simulink model "GyroCLIdent"  (R2021b)
settings: Solver=FixedStepAuto  StartTime=0.0  StopTime=t(end)  FixedStep=Ts  RelTol=1e-3
undefined symbols (not defined in the file): params, x0
libraries: cstblocks x2
settings Model: Creator=Patrick  LastModifiedBy=tom
settings SolverCC: AlgebraicLoopSolver=TrustRegion
settings DebuggingCC: SFMachineParentedDataDiag=warning

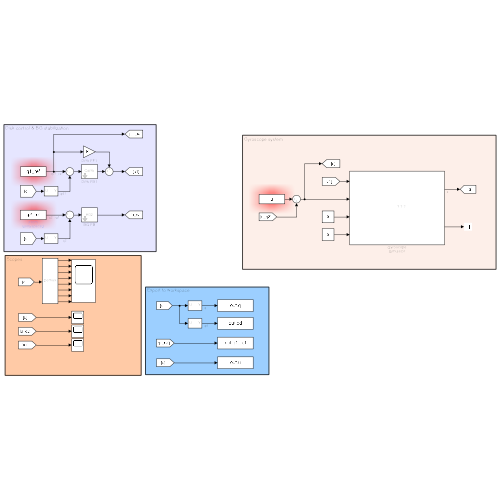
[thumbnail: Simulink's stored preview of the top-level diagram]
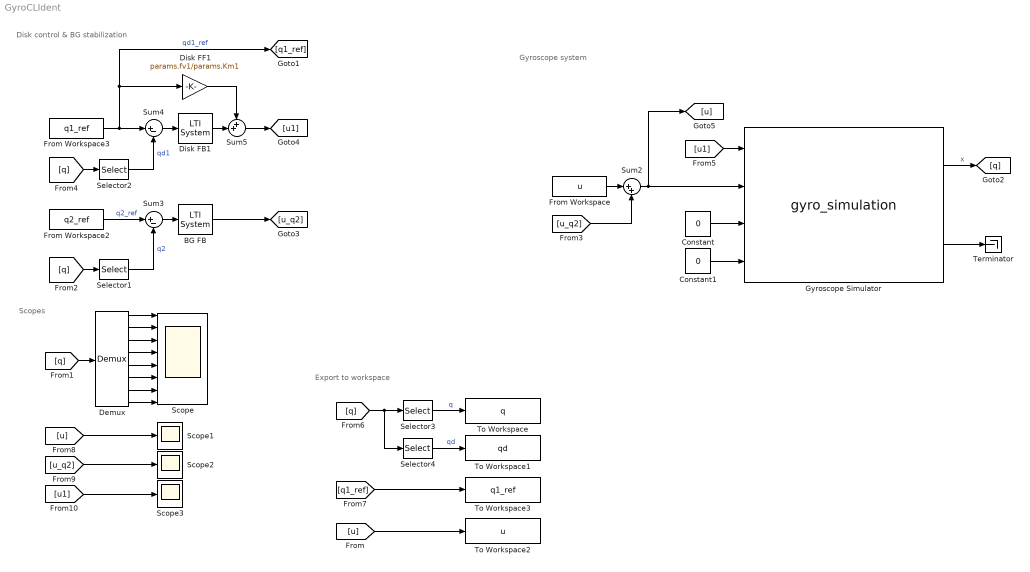
== system GyroCLIdent ==
  note: Gyroscope system
  note: Scopes
  note: Export to workspace
  note: Disk control & BG stabilization
  BG FB : cstblocks/LTI System  sys=Kq2  IC=[]
  Constant : Constant  Value=0
  Constant1 : Constant  Value=0
  Demux : Demux  Outputs=8
      settings: DisplayOption=none
  Disk FB1 : cstblocks/LTI System  sys=Cdisk  IC=[]
  Disk FF1 : Gain  Gain=params.fv1/params.Km1
  From Workspace : FromWorkspace  VariableName=u
  From Workspace2 : FromWorkspace  VariableName=q2_ref
  From Workspace3 : FromWorkspace  VariableName=q1_ref
  Gyroscope Simulator : S-Function  FunctionName=gyro_simulation  Parameters=x0,f,w1l,q2l,q3l,q4l,inertia,Km  SFunctionDeploymentMode=off  EnableBusSupport=off  mask(Gyroscope Simulator){x0=x0, f=[params.fv1;params.fv2;params.fv3;params.fv4], inertia=[params.Ib;params.Ic;params.Id;params.Jb;params.Jc;params.Jd;params.Ka;params.Kb;params.Kc], Km=[params.Km1;params.Km2;params.Km3;params.Km4], w1l=off, q2l=off, q3l=on, q4l=off}
      mask prompts: x0 "Initial conditions (x0):"; f "Viscous friction vector:"; inertia "Inertias:"; Km "Motor constants"; w1l "Disk lock"; q2l "Blue gimbal lock"; q3l "Red gimbal lock"; q4l "Silver gimbal lock"
      mask help:
      | This S-function block simulates the dynamic behavior of the gyroscope setup.
      | Click "Help" for more information.
      mask Help:
      | Outputs are the states of the gyroscope, angular positions and angular velocities, and angles for VRML simulation.
      | The outputs for the states are in the following order:
      | Position disk,
      | Position blue gimbal,
      | Position red gimbal,
      | Position silver gimbal,
      | Velocity disk,
      | Velocity blue gimbal,
      | Velocity red gimbal,
      | Velocity silver gimbal.
      | 
      | Inputs are the torques applied to the following frames:
      | Torque disk,
      | Torque blue gimbal,
      | Torque red gimbal,
      | Torque silver gimbal.
      | 
      | Parameters of the system are the initial conditions "x0" as well as lock options for each frame. The initial conditions should be entered in the same order as the state-outputs are given, seperated by a semicolon.
      | Gyroscope frames can be locked by checking the box for the corresponding frame. In case of locking, the initial conditions can be used to fix a frame under a certain angular position / velocity.
      | 
      | Viscous friction terms can be entered in a [4x1] vector in the order: [disk; blue gimbal; red gimbal; silver gimbal]
      | Inertia parameters can be entered in a [9x1] vector in the order: [Ib;Ic;Id;Jb;Jc;Jd;Ka;Kb;Kc]
      | Motor constants can be entered in a [4x1] vector in the order: [Km1;Km2;Km3;Km4]
      mask DialogControl DescGroupVar Prompt: Gyroscope Simulator
      mask DialogControl DescTextVar Prompt: Simulation block of the Quanser 3 DOF Gyroscope.
      mask DialogControl Gimbal_lock Prompt: Gimbal Lock
      mask Display:
      | disp('dx/dt = f(x,u)\n y = x')
      | image(imread('gyroscope.jpg'))
      | port_label('output',1,'States')
      | port_label('output',2,'VRML')
      | port_label('input',1,'Disk [A]')
      | port_label('input',2,'Bg [A]')
      | port_label('input',3,'Rg [A]')
      | port_label('input',4,'Sg [A]')
  Scope : Scope  NumInputPorts=8
  Scope1 : Scope
  Scope2 : Scope
  Scope3 : Scope
  Selector1 : Selector  InputPortWidth=8  IndexOptions=Index vector (dialog)  Indices=2  OutputSizes=1
  Selector2 : Selector  InputPortWidth=8  IndexOptions=Index vector (dialog)  Indices=5  OutputSizes=1
  Selector3 : Selector  InputPortWidth=8  IndexOptions=Index vector (dialog)  Indices=[1:4]  OutputSizes=1
  Selector4 : Selector  InputPortWidth=8  IndexOptions=Index vector (dialog)  Indices=[5:8]  OutputSizes=1
  Sum2 : Sum  Inputs=|++
  Sum3 : Sum  Inputs=|+-
  Sum4 : Sum  Inputs=|+-
  Sum5 : Sum  Inputs=++|
  Terminator : Terminator
  To Workspace : ToWorkspace  VariableName=q  SaveFormat=Timeseries  SampleTime=-1
  To Workspace1 : ToWorkspace  VariableName=qd  SaveFormat=Timeseries  SampleTime=-1
  To Workspace2 : ToWorkspace  VariableName=u  SaveFormat=Timeseries  SampleTime=-1
  To Workspace3 : ToWorkspace  VariableName=q1_ref  SaveFormat=Timeseries  SampleTime=-1
  wires:
  Gyroscope Simulator/2 -> Terminator/1
  From Workspace/1 -> Sum2/1
  Gyroscope Simulator/1 -> [q]  "x"
  Constant/1 -> Gyroscope Simulator/3
  Constant1/1 -> Gyroscope Simulator/4
  Sum2/1 -> [u], Gyroscope Simulator/2
  [q] -> Selector1/1
  Selector1/1 -> Sum3/2  "q2"
  From Workspace2/1 -> Sum3/1  "q2_ref"
  Sum3/1 -> BG FB/1
  BG FB/1 -> [u_q2]
  From Workspace3/1 -> [q1_ref], Disk FF1/1, Sum4/1  "qd1_ref"
  [q] -> Selector2/1
  Selector2/1 -> Sum4/2  "qd1"
  Sum4/1 -> Disk FB1/1
  Sum5/1 -> [u1]
  Disk FB1/1 -> Sum5/2
  Disk FF1/1 -> Sum5/1
  [u1] -> Gyroscope Simulator/1
  [u_q2] -> Sum2/2
  [q] -> Selector4/1, Selector3/1
  Selector4/1 -> To Workspace1/1  "qd"
  Selector3/1 -> To Workspace/1  "q"
  [q1_ref] -> To Workspace3/1
  [u] -> To Workspace2/1
  Demux/8 -> Scope/8
  Demux/7 -> Scope/7
  Demux/5 -> Scope/5
  Demux/6 -> Scope/6
  Demux/4 -> Scope/4
  Demux/3 -> Scope/3
  Demux/2 -> Scope/2
  Demux/1 -> Scope/1
  [q] -> Demux/1
  [u] -> Scope1/1
  [u_q2] -> Scope2/1
  [u1] -> Scope3/1
